simulink model "EEBL_Scenario_02_cs"  (Simulink 7.6)
settings: Solver=ode5  SolverMode=SingleTasking  StartTime=0.0  StopTime=15  FixedStep=1/100  RelTol=1e-3
model workspace (MAT data in the model file):
  mbox_table : struct (value not decoded)
  model_closed = 0
  sim_status = 0
PreLoadFcn:
  | check_NUTS_defined;
  | 
  | assignin('base',['model_closed_' bdroot],false);addpath('../includes_V2x');
InitFcn:
  | PreScanExperimentInitFcn(bdroot)
StopFcn:
  | PreScanExperimentStopFcn(bdroot)
undefined symbols (not defined in the file): acceleration, actorID, actorType, DiscIntNeverNeededParam, GPS_alt, GPS_lat, GPS_long, intmax, lightBarInUse, messageID, publicVehicleType, rotZ, sireneInUse, trafficLightPriority, turnAdvice, velocity, x_ini_VRML, y_ini_VRML, yawRate, z_ini_VRML
libraries: simulink x54, PreScanSimulinkLibrary x11, simulink_extras x8, PreScanUsefulBlocks x6, simulink_need_slupdate x1
(part 1 of 10)
CloseFcn:
  | evalin('base',['clear model_closed_' bdroot]);
  | 
  | try
  |     close (V2X_PlotSpeed)
  | end
  | 
  | try
  |     close (EEBL_PlotSpeed)
  | end
settings Model: Creator=PRESCAN  LastModifiedBy=buildbot
settings OptimizationCC: InitFltsAndDblsToZero=on
settings DebuggingCC: SaveWithParameterizedLinksMsg=none  SignalResolutionControl=TryResolveAllWithWarning  SolverPrmCheckMsg=none  MultiTaskDSMMsg=warning  MultiTaskCondExecSysMsg=none
settings SFSimCC: SimParseCustomCode=off
settings RTWCC: IncludeERTFirstTime=on
settings GRTTargetCC: TargetFcnLib=ansi_tfl_tmw.mat

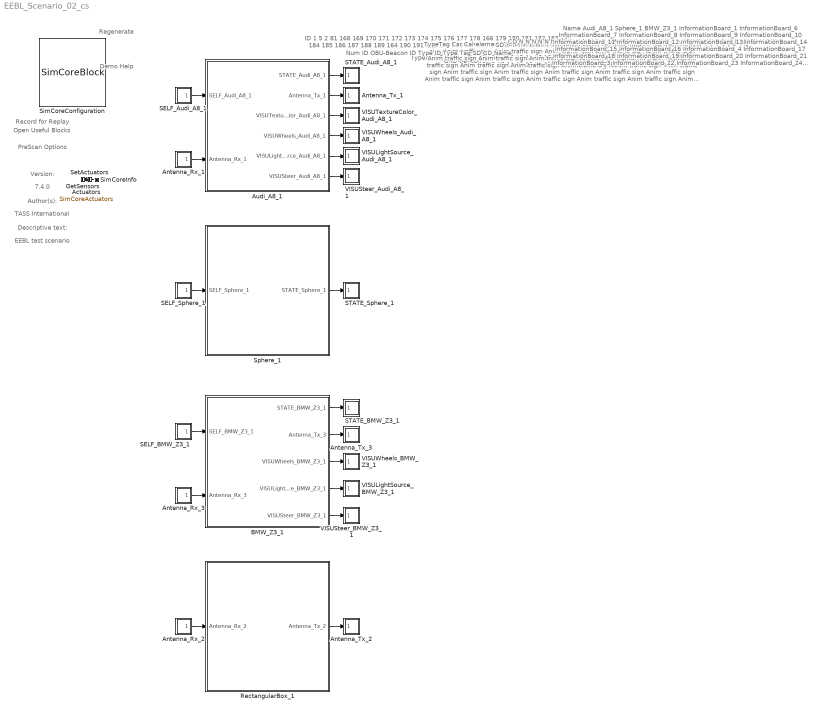
== system EEBL_Scenario_02_cs ==
  note: Demo Help
  note: Regenerate
  note: Record for Replay
  note: Open Useful Blocks
  note: PreScan Options
  note: Version:
  note: 7.4.0
  note: Author(s):
  note: TASS International
  note: Descriptive text:
  note: EEBL test scenario
  note: ID
      |
      | 1
      | 5
      | 2
      | 81
      | 168
      | 169
      | 170
      | 171
      | 172
      | 173
      | 174
      | 175
      | 176
      | 177
      | 178
      | 166
      | 179
      | 180
      | 181
      | 182
      | 183
      | 165
      | 184
      | 185
      | 186
      | 187
      | 188
      | 189
      | 164
      | 190
      | 191
      | 192
      | 193
      | 194
      | 167
      | 195
      | 196
      | 197
      | 198
      | 199
      | 200
      | 201
      | 163
  note: OBU-Beacon ID
  note: TypeID
      |
      | 1
      | 5
      | 1
      | 15
      | 15
      | 15
      | 15
      | 15
      | 15
      | 15
      | 15
      | 15
      | 15
      | 15
      | 15
      | 15
      | 15
      | 15
      | 15
      | 15
      | 15
      | 15
      | 15
      | 15
      | 15
      | 15
      | 15
      | 15
      | 15
      | 15
      | 15
      | 15
      | 15
      | 15
      | 15
      | 15
      | 15
      | 15
      | 15
      | 15
      | 15
      | 15
      | 16
  note: TypeTag
      |
      | Car
      | Cal element
      | Car
      | Anim traffic sign
      | Anim traffic sign
      | Anim traffic sign
      | Anim traffic sign
      | Anim traffic sign
      | Anim traffic sign
      | Anim traffic sign
      | Anim traffic sign
      | Anim traffic sign
      | Anim traffic sign
      | Anim traffic sign
      | Anim traffic sign
      | Anim traffic sign
      | Anim traffic sign
      | Anim traffic sign
      | Anim traffic sign
      | Anim traffic sign
      | Anim traffic sign
      | Anim traffic sign
      | Anim traffic sign
      | Anim traffic sign
      | Anim traffic sign
      | Anim traffic sign
      | Anim traffic sign
      | Anim traffic sign
      | Anim traffic sign
      | Anim traffic sign
      | Anim traffic sign
      | Anim traffic sign
      | Anim traffic sign
      | Anim traffic sign
      | Anim traffic sign
      | Anim traffic sign
      | Anim traffic sign
      | Anim traffic sign
      | Anim traffic sign
      | Anim traffic sign
      | Anim traffic sign
      | Anim traffic sign
      | Abstract object
  note: SD
      |
      | Y
      | Y
      | Y
      | Y
      | Y
      | Y
      | Y
      | Y
      | Y
      | Y
      | Y
      | Y
      | Y
      | Y
      | Y
      | Y
      | Y
      | Y
      | Y
      | Y
      | Y
      | Y
      | Y
      | Y
      | Y
      | Y
      | Y
      | Y
      | Y
      | Y
      | Y
      | Y
      | Y
      | Y
      | Y
      | Y
      | Y
      | Y
      | Y
      | Y
      | Y
      | Y
      | N
  note: CD
      |
      | N
      | N
      | N
      | N
      | N
      | N
      | N
      | N
      | N
      | N
      | N
      | N
      | N
      | N
      | N
      | N
      | N
      | N
      | N
      | N
      | N
      | N
      | N
      | N
      | N
      | N
      | N
      | N
      | N
      | N
      | N
      | N
      | N
      | N
      | N
      | N
      | N
      | N
      | N
      | N
      | N
      | N
      | N
  note: Name
      |
      | Audi_A8_1
      | Sphere_1
      | BMW_Z3_1
      | InformationBoard_1
      | InformationBoard_6
      | InformationBoard_7
      | InformationBoard_8
      | InformationBoard_9
      | InformationBoard_10
      | InformationBoard_11
      | InformationBoard_12
      | InformationBoard_13
      | InformationBoard_14
      | InformationBoard_15
      | InformationBoard_16
      | InformationBoard_4
      | InformationBoard_17
      | InformationBoard_18
      | InformationBoard_19
      | InformationBoard_20
      | InformationBoard_21
      | InformationBoard_3
      | InformationBoard_22
      | InformationBoard_23
      | InformationBoard_24
      | InformationBoard_25
      | InformationBoard_26
      | InformationBoard_27
      | InformationBoard_2
      | InformationBoard_28
      | InformationBoard_29
      | InformationBoard_30
      | InformationBoard_31
      | InformationBoard_32
      | InformationBoard_5
      | InformationBoard_33
      | InformationBoard_34
      | InformationBoard_35
      | InformationBoard_36
      | InformationBoard_37
      | InformationBoard_38
      | InformationBoard_39
      | RectangularBox_1
  note: Num ID OBU-Beacon ID Type ID Type Tag SD CD Name
  Actuators : DataStoreMemory  Tag=Actuators  DataStoreName=SimCoreActuators  InitialValue=zeros(1167,1)
      settings: DeleteFcn=PreScanBlockDeleteFcn;
  Antenna_Rx_1 : Subsystem  Tag=AntennaR  Priority=3  mask(PreScan Source Block: Antenna Receiver){Channel=1, NrEntitiesOut=2, PortName=Antenna_Rx_1, PortIndex=8, PortWidth=456, TimeStep=1/100}
      mask prompts: Channel "User Specified: Channel# [-]"; NrEntitiesOut "User Specified: # of Visible Actors"; PortName "Auto Assigned: Port Name [-]"; PortIndex "Auto Assigned: Index [-]"; PortWidth "Auto Assigned: Port Dimensions [-]"; TimeStep "Auto Assigned: Upload Period [s]"
      mask help:
      | Using the Antenna Receiver (RX) and Transmitter (TX) information between actors can be exchanged. This is done over a channel number to be specified by the user.
      |
      | The Antenna Reciever receives actor information and user-definable signals.
      |
      | For more information, please click Help.
      settings: DeleteFcn=PreScanBlockDeleteFcn;
      mask Help: eval('openHelp(424)')
      mask Display: image(imread('Rx.png'))
  Antenna_Rx_2 : Subsystem  Tag=AntennaR  Priority=3  mask(PreScan Source Block: Antenna Receiver){Channel=1, NrEntitiesOut=2, PortName=Antenna_Rx_2, PortIndex=936, PortWidth=456, TimeStep=1/100}
      mask prompts: Channel "User Specified: Channel# [-]"; NrEntitiesOut "User Specified: # of Visible Actors"; PortName "Auto Assigned: Port Name [-]"; PortIndex "Auto Assigned: Index [-]"; PortWidth "Auto Assigned: Port Dimensions [-]"; TimeStep "Auto Assigned: Upload Period [s]"
      mask help:
      | Using the Antenna Receiver (RX) and Transmitter (TX) information between actors can be exchanged. This is done over a channel number to be specified by the user.
      |
      | The Antenna Reciever receives actor information and user-definable signals.
      |
      | For more information, please click Help.
      settings: DeleteFcn=PreScanBlockDeleteFcn;
      mask Help: eval('openHelp(424)')
      mask Display: image(imread('Rx.png'))
  Antenna_Rx_3 : Subsystem  Tag=AntennaR  Priority=3  mask(PreScan Source Block: Antenna Receiver){Channel=1, NrEntitiesOut=2, PortName=Antenna_Rx_3, PortIndex=480, PortWidth=456, TimeStep=1/100}
      mask prompts: Channel "User Specified: Channel# [-]"; NrEntitiesOut "User Specified: # of Visible Actors"; PortName "Auto Assigned: Port Name [-]"; PortIndex "Auto Assigned: Index [-]"; PortWidth "Auto Assigned: Port Dimensions [-]"; TimeStep "Auto Assigned: Upload Period [s]"
      mask help:
      | Using the Antenna Receiver (RX) and Transmitter (TX) information between actors can be exchanged. This is done over a channel number to be specified by the user.
      |
      | The Antenna Reciever receives actor information and user-definable signals.
      |
      | For more information, please click Help.
      settings: DeleteFcn=PreScanBlockDeleteFcn;
      mask Help: eval('openHelp(424)')
      mask Display: image(imread('Rx.png'))
  Antenna_Tx_1 : Subsystem  Tag=AntennaT  Priority=0  mask(PreScan Sink Block: AntennaT){Channel=1, PortName=Antenna_Tx_1, PortIndex=15, PortWidth=205, TimeStep=1/100}
      mask prompts: Channel "User Specified: Channel# [-]"; PortName "Auto Assigned: Port Name [-]"; PortIndex "Auto Assigned: Index [-]"; PortWidth "Auto Assigned: Port Dimensions [-]"; TimeStep "Auto Assigned: Upload Period [s]"
      mask help:
      | Using the Antenna Receiver (RX) and Transmitter (TX) information between actors can be exchanged. This is done over a channel number to be specified by the user.
      |
      | The Antenna Transmitter contains the following, user-definable signals:
      |
      | - Warning Signal ID	[-]
      | - Maneuvre ID		[-]
      | - Vehicle Type 		[-]
      | - Braking Capacity	[-]
      | - Vehicle Size		[-]
      | - Spares (1:10)		[-]
      |
      | For more information, please click Help.
      settings: DeleteFcn=PreScanBlockDeleteFcn;
      mask Help: eval('openHelp(424)')
      mask Display: image(imread('Tx.png'))
  Antenna_Tx_2 : Subsystem  Tag=AntennaT  Priority=0  mask(PreScan Sink Block: AntennaT){Channel=1, PortName=Antenna_Tx_2, PortIndex=962, PortWidth=205, TimeStep=1/100}
      mask prompts: Channel "User Specified: Channel# [-]"; PortName "Auto Assigned: Port Name [-]"; PortIndex "Auto Assigned: Index [-]"; PortWidth "Auto Assigned: Port Dimensions [-]"; TimeStep "Auto Assigned: Upload Period [s]"
      mask help:
      | Using the Antenna Receiver (RX) and Transmitter (TX) information between actors can be exchanged. This is done over a channel number to be specified by the user.
      |
      | The Antenna Transmitter contains the following, user-definable signals:
      |
      | - Warning Signal ID	[-]
      | - Maneuvre ID		[-]
      | - Vehicle Type 		[-]
      | - Braking Capacity	[-]
      | - Vehicle Size		[-]
      | - Spares (1:10)		[-]
      |
      | For more information, please click Help.
      settings: DeleteFcn=PreScanBlockDeleteFcn;
      mask Help: eval('openHelp(424)')
      mask Display: image(imread('Tx.png'))
  Antenna_Tx_3 : Subsystem  Tag=AntennaT  Priority=0  mask(PreScan Sink Block: AntennaT){Channel=1, PortName=Antenna_Tx_3, PortIndex=481, PortWidth=205, TimeStep=1/100}
      mask prompts: Channel "User Specified: Channel# [-]"; PortName "Auto Assigned: Port Name [-]"; PortIndex "Auto Assigned: Index [-]"; PortWidth "Auto Assigned: Port Dimensions [-]"; TimeStep "Auto Assigned: Upload Period [s]"
      mask help:
      | Using the Antenna Receiver (RX) and Transmitter (TX) information between actors can be exchanged. This is done over a channel number to be specified by the user.
      |
      | The Antenna Transmitter contains the following, user-definable signals:
      |
      | - Warning Signal ID	[-]
      | - Maneuvre ID		[-]
      | - Vehicle Type 		[-]
      | - Braking Capacity	[-]
      | - Vehicle Size		[-]
      | - Spares (1:10)		[-]
      |
      | For more information, please click Help.
      settings: DeleteFcn=PreScanBlockDeleteFcn;
      mask Help: eval('openHelp(424)')
      mask Display: image(imread('Tx.png'))
  Audi_A8_1 : Subsystem  Tag=WorldObjectSubSystem  InitFcn=UniqueId = '13';
      mask Display: image(imread('Audi_A8.jpg'));color('white');text(0,0,' ID=1\n')
  BMW_Z3_1 : Subsystem  Tag=WorldObjectSubSystem  InitFcn=UniqueId = '205';
      mask Display: image(imread('BMW_Z3.jpg'));color('white');text(0,0,' ID=2\n')
  GetSensors : Subsystem  Tag=GetSensors  Priority=2  mask(PreScan Simulation Core Block){NrOfSensors=1392, TimeStep=1/100}
      mask prompts: NrOfSensors "Number of sensor values"; TimeStep "Timestep [s]"
      mask help:
      | Please do not remove this block from the PreScan compilation sheet,
      | as it contains essential configuration parameters for a PreScan simulation.
      settings: DeleteFcn=PreScanBlockDeleteFcn;
  RectangularBox_1 : Subsystem  Tag=WorldObjectSubSystem  InitFcn=UniqueId = '557';
      mask Display: image(imread('RectangularBox.jpg'));color('white');text(0,0,' ID=163\n')
  SELF_Audi_A8_1 : Subsystem  Tag=SELF  Priority=3  mask(PreScan Source Block: SELF){PortName=SELF_Audi_A8_1, PortIndex=0, PortWidth=8, TimeStep=1/100}
      mask prompts: PortName "Auto-Assigned: Port Name [-]"; PortIndex "Auto-Assigned: Port Index [-]"; PortWidth "Auto-Assigned: Port Dimensions"; TimeStep "Auto-Assigned: Upload Period [s]"
      mask help:
      | The SELF port shows (state) information of the actor itself. The outputs are position in the experiment's axis system and the GPS coordinates, and the object's absolute velocity and compass heading.
      |
      | For more information, please click Help.
      settings: DeleteFcn=PreScanBlockDeleteFcn;
      mask Help: eval('openHelp(462)')
      mask Display: image(imread('GPS.png'))
  SELF_BMW_Z3_1 : Subsystem  Tag=SELF  Priority=3  mask(PreScan Source Block: SELF){PortName=SELF_BMW_Z3_1, PortIndex=472, PortWidth=8, TimeStep=1/100}
      mask prompts: PortName "Auto-Assigned: Port Name [-]"; PortIndex "Auto-Assigned: Port Index [-]"; PortWidth "Auto-Assigned: Port Dimensions"; TimeStep "Auto-Assigned: Upload Period [s]"
      mask help:
      | The SELF port shows (state) information of the actor itself. The outputs are position in the experiment's axis system and the GPS coordinates, and the object's absolute velocity and compass heading.
      |
      | For more information, please click Help.
      settings: DeleteFcn=PreScanBlockDeleteFcn;
      mask Help: eval('openHelp(462)')
      mask Display: image(imread('GPS.png'))
  SELF_Sphere_1 : Subsystem  Tag=SELF  Priority=3  mask(PreScan Source Block: SELF){PortName=SELF_Sphere_1, PortIndex=464, PortWidth=8, TimeStep=1/100}
      mask prompts: PortName "Auto-Assigned: Port Name [-]"; PortIndex "Auto-Assigned: Port Index [-]"; PortWidth "Auto-Assigned: Port Dimensions"; TimeStep "Auto-Assigned: Upload Period [s]"
      mask help:
      | The SELF port shows (state) information of the actor itself. The outputs are position in the experiment's axis system and the GPS coordinates, and the object's absolute velocity and compass heading.
      |
      | For more information, please click Help.
      settings: DeleteFcn=PreScanBlockDeleteFcn;
      mask Help: eval('openHelp(462)')
      mask Display: image(imread('GPS.png'))
  STATE_Audi_A8_1 : Subsystem  Tag=State  Priority=0  mask(PreScan Sink Block: State){x0=-2.0003382369952085, y0=3.5736286855864789, z0=0.55, Roll0=0, Pitch0=0, Yaw0=0.92319780373458116, TimeStep=1/100}
      mask prompts: x0 "Ini x-position VEHICLE wrt GLOBAL axis system [m]"; y0 "Ini y-position VEHICLE wrt GLOBAL axis system [m]"; z0 "Ini z-position VEHICLE wrt GLOBAL axis system [m]"; Roll0 "Ini roll-angle BODY wrt VEHICLE axis system [deg]"; Pitch0 "Ini pitch-angle BODY wrt VEHICLE axis system [deg]"; Yaw0 "Ini yaw-angle VEHICLE wrt GLOBAL axis system [deg]"; TimeStep "Time Step [s]"
      mask help:
      | The Actor State contains a vector signal of size (9x1), containing the following signals:
      |
      | -  Position                  (x,y,z)                                     [m]
      | -  Velocity                  (vx,vy,vz)                               [m/s]
      | -  Angles                    (Roll, Pitch, Yaw)                   [rad]
      |
      | The Actor state is defined in the global axis system.
      | The state is superponed on the Initial position defined in the GUI.
      |
      | For more information, please click Help.
      settings: DeleteFcn=PreScanBlockDeleteFcn;
      mask Help: eval('openHelp(222)')
      mask Display: image(imread('State.png'))
  STATE_BMW_Z3_1 : Subsystem  Tag=State  Priority=0  mask(PreScan Sink Block: State){x0=59.766689592078251, y0=8.4452137651818937, z0=0.69, Roll0=0, Pitch0=0, Yaw0=8.0780561606359811, TimeStep=1/100}
      mask prompts: x0 "Ini x-position VEHICLE wrt GLOBAL axis system [m]"; y0 "Ini y-position VEHICLE wrt GLOBAL axis system [m]"; z0 "Ini z-position VEHICLE wrt GLOBAL axis system [m]"; Roll0 "Ini roll-angle BODY wrt VEHICLE axis system [deg]"; Pitch0 "Ini pitch-angle BODY wrt VEHICLE axis system [deg]"; Yaw0 "Ini yaw-angle VEHICLE wrt GLOBAL axis system [deg]"; TimeStep "Time Step [s]"
      mask help:
      | The Actor State contains a vector signal of size (9x1), containing the following signals:
      |
      | -  Position                  (x,y,z)                                     [m]
      | -  Velocity                  (vx,vy,vz)                               [m/s]
      | -  Angles                    (Roll, Pitch, Yaw)                   [rad]
      |
      | The Actor state is defined in the global axis system.
      | The state is superponed on the Initial position defined in the GUI.
      |
      | For more information, please click Help.
      settings: DeleteFcn=PreScanBlockDeleteFcn;
      mask Help: eval('openHelp(222)')
      mask Display: image(imread('State.png'))
  STATE_Sphere_1 : Subsystem  Tag=State  Priority=0  mask(PreScan Sink Block: State){x0=-2.0003746851196036, y0=3.5683845581685842, z0=0, Roll0=0, Pitch0=0, Yaw0=0.65951613396799758, TimeStep=1/100}
      mask prompts: x0 "Ini x-position VEHICLE wrt GLOBAL axis system [m]"; y0 "Ini y-position VEHICLE wrt GLOBAL axis system [m]"; z0 "Ini z-position VEHICLE wrt GLOBAL axis system [m]"; Roll0 "Ini roll-angle BODY wrt VEHICLE axis system [deg]"; Pitch0 "Ini pitch-angle BODY wrt VEHICLE axis system [deg]"; Yaw0 "Ini yaw-angle VEHICLE wrt GLOBAL axis system [deg]"; TimeStep "Time Step [s]"
      mask help:
      | The Actor State contains a vector signal of size (9x1), containing the following signals:
      |
      | -  Position                  (x,y,z)                                     [m]
      | -  Velocity                  (vx,vy,vz)                               [m/s]
      | -  Angles                    (Roll, Pitch, Yaw)                   [rad]
      |
      | The Actor state is defined in the global axis system.
      | The state is superponed on the Initial position defined in the GUI.
      |
      | For more information, please click Help.
      settings: DeleteFcn=PreScanBlockDeleteFcn;
      mask Help: eval('openHelp(222)')
      mask Display: image(imread('State.png'))
  SetActuators : Subsystem  Tag=SetActuators  Priority=1  mask(PreScan Simulation Core Block){TimeStep=1/100, NrOfActuators=1167}
      mask prompts: TimeStep "Timestep [s]"; NrOfActuators "Number of actuator values"
      mask help:
      | Please do not remove this block from the PreScan compilation sheet,
      | as it contains essential configuration parameters for a PreScan simulation.
      settings: DeleteFcn=PreScanBlockDeleteFcn;
  SimCoreConfiguration : M-S-Function  Tag=SimCoreConfiguration  Description=7554E7A75508BA4AB74C9CE496844D0A64444FB1F4C419A76FFCA00764D87D8D  FunctionName=SimCoreBlock  Parameters=ExperimentXML PortsXML SimulationCore HostName CheckStart EnableLog RfR EnableGPUAccel ShowComputationTime  mask(PreScan Simulation Core Configurator){SimulationCore=NUTS, HostName=0, CheckStart=0, prescanversion='7.4.0', EnableLog=off, RfR=0, EnableGPUAccel=off, ShowComputationTime=off}
      mask prompts: SimulationCore "Simulation Core"; HostName "Simulation Host"; CheckStart "Show START Dialog"; prescanversion "PreScan Version"; EnableLog "Create TA Log"; RfR "Record for Replay"; EnableGPUAccel "Enable GPU Acceleration"; ShowComputationTime "Show ComputationTime Scope"
      mask help:
      | Please do not remove this block from the PreScan compilation sheet,
      | as it contains essential configuration parameter for a PreScan simulation.
      mask init:
      | model = bdroot;
      | ExperimentXML = [model(1:end-3) '.pex'];
      | PortsXML = [model '_ports.pcd'];
      settings: DeleteFcn=PreScanBlockDeleteFcn;  ModelCloseFcn=assignin('base',['model_closed_' bdroot],true);
      mask Help: eval('openHelp(812)')
      mask Display: image(imread('prescanlogo.ico'))
  SimCoreInfo : Subsystem  Tag=SimCoreInfo
  Sphere_1 : Subsystem  Tag=WorldObjectSubSystem  InitFcn=UniqueId = '36';
      mask Display: image(imread('Sphere.jpg'));color('white');text(0,0,' ID=5\n')
  VISULightSource_Audi_A8_1 : Subsystem  Tag=VisuLightSource  Priority=0
      settings: DeleteFcn=PreScanBlockDeleteFcn;
      mask Type: PreScan Sink Block: VisuLightSource
      mask Description:
      | The VisuLightSource block provides a way to animate Light Sources of the indicator, braking, fog and main lights of a vehicle.
      | 
      | For more information, please click Help.
      mask Help: eval('openHelp(223)')
      mask Display: image(imread('RearLight.png'))
  VISULightSource_BMW_Z3_1 : Subsystem  Tag=VisuLightSource  Priority=0
      settings: DeleteFcn=PreScanBlockDeleteFcn;
      mask Type: PreScan Sink Block: VisuLightSource
      mask Description:
      | The VisuLightSource block provides a way to animate Light Sources of the indicator, braking, fog and main lights of a vehicle.
      | 
      | For more information, please click Help.
      mask Help: eval('openHelp(223)')
      mask Display: image(imread('RearLight.png'))
  VISUSteer_Audi_A8_1 : Subsystem  Tag=VisuSteer  Priority=0
      settings: DeleteFcn=PreScanBlockDeleteFcn;
      mask Type: PreScan Sink Block: VisuSteer
      mask Description:
      | The VisuSteer block provides a way to adapt the orientation of the steering column and steering wheel of a vehicle.
      | 
      | For more information, please click Help.
      mask Help: eval('openHelp(223)')
      mask Display: image(imread('steeringwheel.png'))
  VISUSteer_BMW_Z3_1 : Subsystem  Tag=VisuSteer  Priority=0
      settings: DeleteFcn=PreScanBlockDeleteFcn;
      mask Type: PreScan Sink Block: VisuSteer
      mask Description:
      | The VisuSteer block provides a way to adapt the orientation of the steering column and steering wheel of a vehicle.
      | 
      | For more information, please click Help.
      mask Help: eval('openHelp(223)')
      mask Display: image(imread('steeringwheel.png'))
  VISUTextureColor_Audi_A8_1 : Subsystem  Tag=VisuTextureColor  Priority=0
      settings: DeleteFcn=PreScanBlockDeleteFcn;
      mask Type: PreScan Sink Block: VisuTextureColor
      mask Description:
      | The Texture Color block provides a way to adapt the color of a vehicle.
      | 
      | For more information, please click Help.
      mask Help: eval('openHelp(230)')
      mask Display: image(imread('TextureColor.png'))
  VISUWheels_Audi_A8_1 : Subsystem  Tag=VisuWheels  Priority=0
      settings: DeleteFcn=PreScanBlockDeleteFcn;
      mask Type: PreScan Sink Block: VisuWheels
      mask Description:
      | The VisuWheels block provides a way to animate the wheels of a vehicle, with steering, rotation (because of velocity) and z-displacement.
      | 
      | For more information, please click Help.
      mask Help: eval('openHelp(223)')
      mask Display: image(imread('wheel.png'))
  VISUWheels_BMW_Z3_1 : Subsystem  Tag=VisuWheels  Priority=0
      settings: DeleteFcn=PreScanBlockDeleteFcn;
      mask Type: PreScan Sink Block: VisuWheels
      mask Description:
      | The VisuWheels block provides a way to animate the wheels of a vehicle, with steering, rotation (because of velocity) and z-displacement.
      | 
      | For more information, please click Help.
      mask Help: eval('openHelp(223)')
      mask Display: image(imread('wheel.png'))
  wires:
  Audi_A8_1/1(STATE_Audi_A8_1) -> STATE_Audi_A8_1/1(State)
  SELF_Audi_A8_1/1(U) -> Audi_A8_1/1(SELF_Audi_A8_1)
  Antenna_Rx_1/1(U) -> Audi_A8_1/2(Antenna_Rx_1)
  Audi_A8_1/2(Antenna_Tx_1) -> Antenna_Tx_1/1(Y)
  Audi_A8_1/3(VISUTextureColor_Audi_A8_1) -> VISUTextureColor_Audi_A8_1/1(TextureColor)
  Audi_A8_1/4(VISUWheels_Audi_A8_1) -> VISUWheels_Audi_A8_1/1(Wheels)
  Audi_A8_1/5(VISULightSource_Audi_A8_1) -> VISULightSource_Audi_A8_1/1(Lights)
  Audi_A8_1/6(VISUSteer_Audi_A8_1) -> VISUSteer_Audi_A8_1/1(Steer)
  Sphere_1/1(STATE_Sphere_1) -> STATE_Sphere_1/1(State)
  SELF_Sphere_1/1(U) -> Sphere_1/1(SELF_Sphere_1)
  BMW_Z3_1/1(STATE_BMW_Z3_1) -> STATE_BMW_Z3_1/1(State)
  SELF_BMW_Z3_1/1(U) -> BMW_Z3_1/1(SELF_BMW_Z3_1)
  Antenna_Rx_3/1(U) -> BMW_Z3_1/2(Antenna_Rx_3)
  BMW_Z3_1/2(Antenna_Tx_3) -> Antenna_Tx_3/1(Y)
  BMW_Z3_1/3(VISUWheels_BMW_Z3_1) -> VISUWheels_BMW_Z3_1/1(Wheels)
  BMW_Z3_1/4(VISULightSource_BMW_Z3_1) -> VISULightSource_BMW_Z3_1/1(Lights)
  BMW_Z3_1/5(VISUSteer_BMW_Z3_1) -> VISUSteer_BMW_Z3_1/1(Steer)
  Antenna_Rx_2/1(U) -> RectangularBox_1/1(Antenna_Rx_2)
  RectangularBox_1/1(Antenna_Tx_2) -> Antenna_Tx_2/1(Y)
  SetActuators/1(dummy) -> GetSensors/1(dummy)

== system EEBL_Scenario_02_cs/Antenna_Rx_1 ==
  Selector : Selector  IndexMode=Zero-based  IndexOptions=Starting index (dialog)  Indices=PortIndex  OutputSizes=PortWidth(1)
  U : Outport
  wires:
  Selector/1 -> U/1
  [SimCoreSensors] -> Selector/1

== system EEBL_Scenario_02_cs/Antenna_Rx_2 ==
  Selector : Selector  IndexMode=Zero-based  IndexOptions=Starting index (dialog)  Indices=PortIndex  OutputSizes=PortWidth(1)
  U : Outport
  wires:
  Selector/1 -> U/1
  [SimCoreSensors] -> Selector/1

== system EEBL_Scenario_02_cs/Antenna_Rx_3 ==
  Selector : Selector  IndexMode=Zero-based  IndexOptions=Starting index (dialog)  Indices=PortIndex  OutputSizes=PortWidth(1)
  U : Outport
  wires:
  Selector/1 -> U/1
  [SimCoreSensors] -> Selector/1

== system EEBL_Scenario_02_cs/Antenna_Tx_1 ==
  Y : Inport
  Assignment : Assignment  IndexMode=Zero-based  SampleTime=TimeStep  IndexOptions=Starting index (dialog)  Indices=PortIndex  OutputSizes=[1 1]
  Data Store Read : DataStoreRead  DataStoreName=SimCoreActuators  SampleTime=TimeStep
  Data Store Write : DataStoreWrite  DataStoreName=SimCoreActuators
  wires:
  Assignment/1 -> Data Store Write/1
  Data Store Read/1 -> Assignment/1
  Y/1 -> Assignment/2

== system EEBL_Scenario_02_cs/Antenna_Tx_2 ==
  Y : Inport
  Assignment : Assignment  IndexMode=Zero-based  SampleTime=TimeStep  IndexOptions=Starting index (dialog)  Indices=PortIndex  OutputSizes=[1 1]
  Data Store Read : DataStoreRead  DataStoreName=SimCoreActuators  SampleTime=TimeStep
  Data Store Write : DataStoreWrite  DataStoreName=SimCoreActuators
  wires:
  Assignment/1 -> Data Store Write/1
  Data Store Read/1 -> Assignment/1
  Y/1 -> Assignment/2

== system EEBL_Scenario_02_cs/Antenna_Tx_3 ==
  Y : Inport
  Assignment : Assignment  IndexMode=Zero-based  SampleTime=TimeStep  IndexOptions=Starting index (dialog)  Indices=PortIndex  OutputSizes=[1 1]
  Data Store Read : DataStoreRead  DataStoreName=SimCoreActuators  SampleTime=TimeStep
  Data Store Write : DataStoreWrite  DataStoreName=SimCoreActuators
  wires:
  Assignment/1 -> Data Store Write/1
  Data Store Read/1 -> Assignment/1
  Y/1 -> Assignment/2

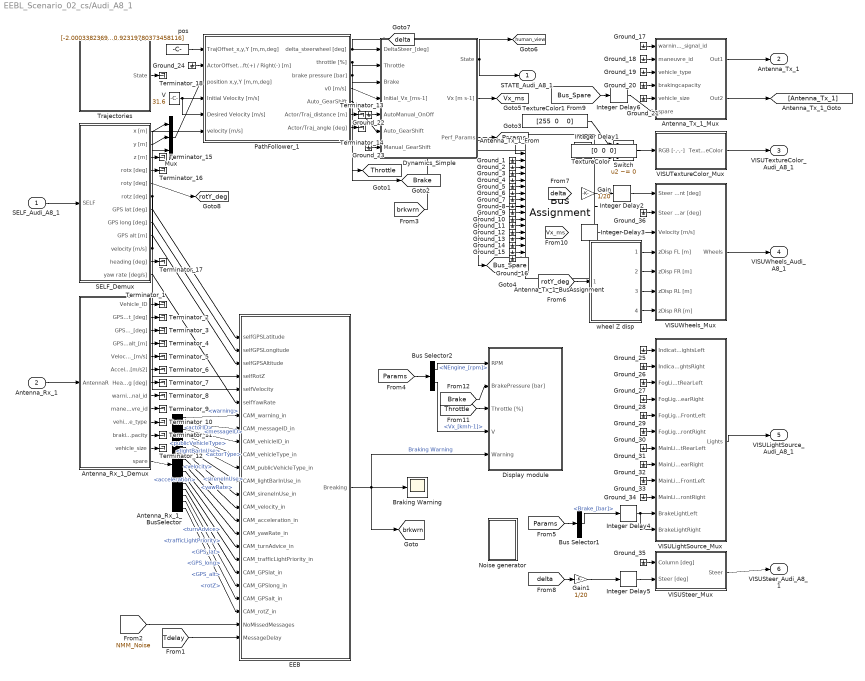
== system EEBL_Scenario_02_cs/Audi_A8_1 ==
  SELF_Audi_A8_1 : Inport  Tag=SELFInport
  Antenna_Rx_1 : Inport  Tag=AntennaRInport  Port=2
  Antenna_Rx_1_BusSelector : BusSelector  Tag=BusAntennaR  OutputSignals=warning,messageID,actorID,actorType,publicVehicleType,lightBarInUse,sireneInUse,velocity,acceleration,yawRate,turnAdvice,trafficLightPriority,GPS_lat,GPS_long,GPS_alt,rotZ
  Antenna_Rx_1_Demux : Subsystem  Tag=DemuxAntennaR  mask(PreScan Demux Block:){Channel=1}
      settings: DeleteFcn=PreScanBlockDeleteFcn;
      mask Display:
      | fprintf('Channel: %d',Channel)
      | port_label('output', 1, 'Vehicle_ID')
      | port_label('output', 2, 'GPS Pos Lat [deg]')
      | port_label('output', 3, 'GPS Pos Long [deg]')
      | port_label('output', 4, 'GPS Pos Alt [m]')
      | port_label('output', 5, 'Velocity [m/s]')
      | port_label('output', 6, 'Acceleration [m/s2]')
      | port_label('output', 7, 'Heading [deg]')
      | port_label('output', 8, 'Warning signal ID')
      | port_label('output', 9, 'Maneuvre ID')
      | port_label('output', 10, 'Vehicle Type')
      | port_label('output', 11, 'Braking Capacity')
      | port_label('output', 12, 'Vehicle Size')
      | port_label('output', 13, 'Spare')
  Antenna_Tx_1_BusAssignment : BusAssignment  Tag=BusAntennaT  AssignedSignals=warning,messageID,actorID,actorType,publicVehicleType,lightBarInUse,sireneInUse,velocity,acceleration,yawRate,turnAdvice,trafficLightPriority,GPS_lat,GPS_long,GPS_alt,rotZ
  Antenna_Tx_1_Mux : Subsystem  Tag=MuxAntennaT  mask(PreScan Mux Block:){Channel=1, TimeStep=1/100}
      mask prompts: TimeStep "Time Step [s]"
      settings: DeleteFcn=PreScanBlockDeleteFcn;
      mask Display:
      | fprintf('Channel: %d',Channel)
      | port_label('input', 1, 'Warning signal ID')
      | port_label('input', 2, 'Maneuvre ID')
      | port_label('input', 3, 'Vehicle Type')
      | port_label('input', 4, 'Braking Capacity')
      | port_label('input', 5, 'Vehicle Size')
      | port_label('input', 6, 'spare')
  Braking Warning : Scope
      settings: SaveName=ScopeData2
  Bus Selector1 : BusSelector  OutputSignals=Brake_[bar]
  Bus Selector2 : BusSelector  OutputSignals=NEngine_[rpm],Vx_[kmh-1]
  Display module : Subsystem  mask{DisplaySwitch=on, DisplayFreq=25}
      mask prompts: DisplaySwitch "Dispaly"; DisplayFreq "Display Frequency"
  Dynamics_Simple : Subsystem  Tag=Simple_Vehicle_Dynamics  mask(PreScan Block: Simple Dynamics){Migrate=off, TimeStep=1/100, ComputationMode=Continuous_Time}
      mask prompts: Migrate "Migrate. During migration this block will be replaced by a newer one."; TimeStep "Auto assigned: Time Step [s]"; ComputationMode "Computation mode:"
      mask help:
      | The Simple Dynamics Model is selected in the GUI to simulate vehicle dynamics behavior.
      |
      | The Simple Dynamics Model is completely open to the user. The parameters of this model can be set in the Simple Dynamics dialog in the GUI.
      |
      | For more information, please click Help.
      mask init:
      | p = SimpleDyn_pars;
      settings: DeleteFcn=PreScanBlockDeleteFcn;
      mask Help: eval('openHelp(220)')
      mask Display:
      | image(imread('SimpleDyn.png'))
      | port_label('input', 1, '{\delta}_S_t_ _e_e_r [deg]','texmode','on')
      | port_label('input', 2, 'Throttle [%]')
      | port_label('input', 3, 'Brake Pres [bar]')
      | port_label('input', 4, 'V_0 [ms-1]','texmode','on')
      | port_label('input', 5, 'Auto=[0]/Manual=[1]')
      | port_label('input', 6, 'Auto_GearShift')
      | port_label('input', 7, 'Manual_GearShift')
      | port_label('output', 1, 'State')
      | port_label('output', 2, 'Vx [ms-1]')
      | port_label('output', 3, 'Perf Params')
  EEB : Subsystem
  Gain : Gain  Gain=1/20
  Gain1 : Gain  Gain=1/20
  Ground_{1..36} (36 alike) : Ground
  Integer Delay{1..6} (6 alike) : simulink/Discrete/Integer Delay  NumDelays=1  InputProcessing=Inherited  vinit=0.0  samptime=-1
  Mux : Mux  Inputs=3
  Noise generator : Subsystem
  PathFollower_1 : Subsystem  Tag=pathFollower  mask(PreScan Block: Path Follower){Migrate=on, FileName='Trajectory_1.mat', TunableSteeringGain=1, XShifting_wrt_COG=0}
      mask prompts: Migrate "Migrate. During migration this block will be replaced by a newer one."; FileName "Trajectory Name"; TunableSteeringGain "TunableSteeringGain [-]"; XShifting_wrt_COG "XShifting_wrt_COG [m]"
      mask help:
      | The Path Follower Model is selected in the GUI to simulate driver behavior.
      |
      | For more information, please click Help.
      mask init:
      | load(['trajectories/',eval(FileName)])
      | traject=trajectory';
      | 
      | Traj_x=traject(:,2);
      | Traj_y=traject(:,3);
      | Traj_z=traject(:,4);
      | Traj_vx=traject(:,8);
      | Traj_vy=traject(:,9);
      | Traj_vz=traject(:,10);
      mask Help: eval('openHelp(232)')
  SELF_Demux : Subsystem  Tag=DemuxSELF
      settings: DeleteFcn=PreScanBlockDeleteFcn;
      mask Type: PreScan Demux Block:
      mask Display:
      | port_label('output',1,'x [m]')
      | port_label('output',2,'y [m]')
      | port_label('output',3,'z [m]','texmode','on')
      | port_label('output',4,'Rotx [deg]','texmode','on')
      | port_label('output',5,'Roty [deg]','texmode','on')
      | port_label('output',6,'Rotz [deg]','texmode','on')
      | port_label('output',7,'GPS lat [deg]','texmode','on')
      | port_label('output',8,'GPS long [deg]','texmode','on')
      | port_label('output',9,'GPS alt [m]','texmode','on')
      | port_label('output',10,'Velocity [m/s]')
      | port_label('output',11,'Heading [deg]')
      | port_label('output',12,'Yaw rate [deg/s]')
  Switch : Switch  Criteria=u2 ~= 0
  Terminator_{1..18} (18 alike) : Terminator
  TextureColor : Constant  Tag=TextureColor  Value="[0  0  0]"
  TextureColor1 : Constant  Tag=TextureColor  Value="[255  0    0]"
  Trajectories : Subsystem  Tag=Trajectories
      settings: DeleteFcn=PreScanBlockDeleteFcn;
      mask Type: PreScan Source Block: Trajectories
      mask Description:
      | The Trajectory block contains the trajectories defined in the PreScan Experiment Editor. The output of the trajectory block is the (vehicle) State.
      | 
      | For more information, please click Help.
      mask Help: eval('openHelp(312)')
      mask Display: image(imread('Trajectory.png'));
  V : Constant  Value=31.6
  VISULightSource_Mux : Subsystem  Tag=MuxLightSource
      settings: DeleteFcn=PreScanBlockDeleteFcn;
      mask Type: PreScan Mux Block:
  VISUSteer_Mux : Subsystem  Tag=MuxSteer
      settings: DeleteFcn=PreScanBlockDeleteFcn;
      mask Type: PreScan Mux Block:
  VISUTextureColor_Mux : Subsystem  Tag=MuxSteer
      settings: DeleteFcn=PreScanBlockDeleteFcn;
      mask Type: PreScan Mux Block:
  VISUWheels_Mux : Subsystem  Tag=MuxWheels  mask(PreScan Mux Block:){TimeStep=1/100}
      mask prompts: TimeStep "Auto Assigned: Time Step [s]"
      settings: DeleteFcn=PreScanBlockDeleteFcn;
  pos : Constant  Tag=pos  Value=[-2.0003382369952085 3.5736286855864789 0.92319780373458116]
  wheel Z disp : Subsystem  mask(Simple Dynamics parameters){a=1.17, b=1.77}
      mask prompts: a "Distance to the front wheel from cars center of gravity a [m]"; b "Distance to the back wheel from cars center of gravity b [m]"
  STATE_Audi_A8_1 : Outport  Tag=StateOutport
  Antenna_Tx_1 : Outport  Tag=AntennaTOutport  Port=2
  VISUTextureColor_Audi_A8_1 : Outport  Tag=VisuTextureColorOutport  Port=3  SampleTime=1/100
  VISUWheels_Audi_A8_1 : Outport  Tag=VisuWheelsOutport  Port=4  SampleTime=1/100
  VISULightSource_Audi_A8_1 : Outport  Tag=VisuLightsOutport  Port=5  SampleTime=1/100
  VISUSteer_Audi_A8_1 : Outport  Tag=VisuSteerOutport  Port=6  SampleTime=1/100
  tag scope: Brake=global, Bus_Spare=global, Params=global, Throttle=global, Vx_ms=global, brkwrn=global, delta=global, human_view=global, rotY_deg=global
  wires:
  [delta] -> Gain/1
  [rotY_deg] -> wheel Z disp/1(rotY [deg])
  [NMM_Noise] -> EEB/23(NoMissedMessages)
  [Tdelay] -> EEB/24(MessageDelay)
  EEB/1(Breaking) -> Braking Warning/1, [brkwrn], Display module/5(Warning)  "Braking Warning"
  [brkwrn] -> Integer Delay1/1
  Gain/1 -> Integer Delay2/1
  [Bus_Spare] -> Integer Delay6/1
  Integer Delay1/1 -> Switch/2
  [Vx_ms] -> Integer Delay3/1
  [delta] -> Gain1/1
  Bus Selector1/1 -> Integer Delay4/1  "<Brake_[bar]>"
  Gain1/1 -> Integer Delay5/1
  [Params] -> Bus Selector1/1
  Bus Selector2/1 -> Display module/1(RPM)  "<NEngine_[rpm]>"
  Bus Selector2/2 -> Display module/4(V)  "<Vx_[kmh-1]>"
  [Params] -> Bus Selector2/1
  [Throttle] -> Display module/3(Throttle [%])
  [Brake] -> Display module/2(BrakePressure [bar])
  pos/1 -> PathFollower_1/1(TrajOffset_x,y,Y [m,m,deg])
  SELF_Audi_A8_1/1 -> SELF_Demux/1(SELF)
  Antenna_Rx_1_Demux/13(spare) -> Antenna_Rx_1_BusSelector/1
  Antenna_Rx_1/1 -> Antenna_Rx_1_Demux/1(AntennaR)
  Antenna_Tx_1_Mux/2(Out2) -> [Antenna_Tx_1]
  [Antenna_Tx_1] -> Antenna_Tx_1_BusAssignment/1
  Antenna_Tx_1_Mux/1(Out1) -> Antenna_Tx_1/1
  VISUTextureColor_Mux/1(TextureColor) -> VISUTextureColor_Audi_A8_1/1
  TextureColor/1 -> Switch/3
  VISUWheels_Mux/1(Wheels) -> VISUWheels_Audi_A8_1/1
  VISULightSource_Mux/1(Lights) -> VISULightSource_Audi_A8_1/1
  VISUSteer_Mux/1(Steer) -> VISUSteer_Audi_A8_1/1
  Dynamics_Simple/2(Vx [m s-1]) -> [Vx_ms]
  PathFollower_1/4(v0 [m/s]) -> Dynamics_Simple/4(Initial_Vx_[ms-1])
  PathFollower_1/5(Auto_GearShift) -> Dynamics_Simple/6(Auto_GearShift)
  PathFollower_1/1(delta_steerwheel [deg]) -> Dynamics_Simple/1(DeltaSteer_[deg]), [delta]
  Dynamics_Simple/1(State) -> STATE_Audi_A8_1/1, [human_view]
  Antenna_Rx_1_BusSelector/16 -> EEB/22(CAM_rotZ_in)  "<rotZ>"
  Antenna_Rx_1_BusSelector/15 -> EEB/21(CAM_GPSalt_in)  "<GPS_alt>"
  Antenna_Rx_1_BusSelector/14 -> EEB/20(CAM_GPSlong_in)  "<GPS_long>"
  Antenna_Rx_1_BusSelector/13 -> EEB/19(CAM_GPSlat_in)  "<GPS_lat>"
  Antenna_Rx_1_BusSelector/12 -> EEB/18(CAM_trafficLightPriority_in)  "<trafficLightPriority>"
  Antenna_Rx_1_BusSelector/11 -> EEB/17(CAM_turnAdvice_in)  "<turnAdvice>"
  Antenna_Rx_1_BusSelector/10 -> EEB/16(CAM_yawRate_in)  "<yawRate>"
  Antenna_Rx_1_BusSelector/9 -> EEB/15(CAM_acceleration_in)  "<acceleration>"
  Antenna_Rx_1_BusSelector/8 -> EEB/14(CAM_velocity_in)  "<velocity>"
  Antenna_Rx_1_BusSelector/7 -> EEB/13(CAM_sireneInUse_in)  "<sireneInUse>"
  Antenna_Rx_1_BusSelector/6 -> EEB/12(CAM_lightBarInUse_in)  "<lightBarInUse>"
  Antenna_Rx_1_BusSelector/5 -> EEB/11(CAM_publicVehicleType_in)  "<publicVehicleType>"
  Antenna_Rx_1_BusSelector/4 -> EEB/10(CAM_vehicleType_in)  "<actorType>"
  Antenna_Rx_1_BusSelector/3 -> EEB/9(CAM_vehicleID_in)  "<actorID>"
  Antenna_Rx_1_BusSelector/2 -> EEB/8(CAM_messageID_in)  "<messageID>"
  Antenna_Rx_1_BusSelector/1 -> EEB/7(CAM_warning_in)  "<warning>"
  SELF_Demux/9(GPS alt [m]) -> EEB/3(selfGPSAltitude)
  SELF_Demux/8(GPS long [deg]) -> EEB/2(selfGPSLongitude)
  SELF_Demux/7(GPS lat [deg]) -> EEB/1(selfGPSLatitude)
  PathFollower_1/3(brake pressure [bar]) -> Dynamics_Simple/3(Brake), [Brake]
  PathFollower_1/2(throttle [%]) -> Dynamics_Simple/2(Throttle), [Throttle]
  SELF_Demux/12(yaw rate [deg/s]) -> EEB/6(selfYawRate)
  SELF_Demux/5(roty [deg]) -> [rotY_deg]
  wheel Z disp/4(zDisp RR [m]) -> VISUWheels_Mux/7(zDisp RR [m])
  wheel Z disp/3(zDisp RL [m]) -> VISUWheels_Mux/6(zDisp RL [m])
  wheel Z disp/2(zDisp FR [m]) -> VISUWheels_Mux/5(zDisp FR [m])
  wheel Z disp/1(zDisp FL [m]) -> VISUWheels_Mux/4(zDisp FL [m])
  SELF_Demux/10(velocity [m/s]) -> PathFollower_1/6(velocity [m/s]), EEB/5(selfVelocity)
  SELF_Demux/6(rotz [deg]) -> Mux/3, EEB/4(selfRotZ)
  SELF_Demux/2(y [m]) -> Mux/2
  SELF_Demux/1(x [m]) -> Mux/1
  Mux/1 -> PathFollower_1/3(position x,y,Y [m,m,deg])
  V/1 -> PathFollower_1/4(Initial Velocity [m/s]), PathFollower_1/5(Desired Velocity [m/s])
  TextureColor1/1 -> Switch/1
  Switch/1 -> VISUTextureColor_Mux/1(RGB [-,-,-])
  Integer Delay6/1 -> Antenna_Tx_1_Mux/6(spare)
  Integer Delay2/1 -> VISUWheels_Mux/1(Steer Angle Front [deg])
  Dynamics_Simple/3(Perf_Params) -> [Params]
  Integer Delay3/1 -> VISUWheels_Mux/3(Velocity [m/s])
  Integer Delay4/1 -> VISULightSource_Mux/11(BrakeLightLeft), VISULightSource_Mux/12(BrakeLightRight)
  Integer Delay5/1 -> VISUSteer_Mux/2(Steer [deg])
  Antenna_Tx_1_BusAssignment/1 -> [Bus_Spare]
  Antenna_Rx_1_Demux/1(Vehicle_ID) -> Terminator_1/1
  Antenna_Rx_1_Demux/2(GPS_pos_lat_[deg]) -> Terminator_2/1
  Antenna_Rx_1_Demux/3(GPS_pos_long_[deg]) -> Terminator_3/1
  Antenna_Rx_1_Demux/4(GPS_pos_alt_[m]) -> Terminator_4/1
  Antenna_Rx_1_Demux/5(Velocity_[m/s]) -> Terminator_5/1
  Antenna_Rx_1_Demux/6(Acceleration_[m/s2]) -> Terminator_6/1
  Antenna_Rx_1_Demux/7(Heading [deg]) -> Terminator_7/1
  Antenna_Rx_1_Demux/8(warning_signal_id) -> Terminator_8/1
  Antenna_Rx_1_Demux/9(maneuvre_id) -> Terminator_9/1
  Antenna_Rx_1_Demux/10(vehicle_type) -> Terminator_10/1
  Antenna_Rx_1_Demux/11(brakingcapacity) -> Terminator_11/1
  Antenna_Rx_1_Demux/12(vehicle_size) -> Terminator_12/1
  Ground_1/1 -> Antenna_Tx_1_BusAssignment/2
  Ground_2/1 -> Antenna_Tx_1_BusAssignment/3
  Ground_3/1 -> Antenna_Tx_1_BusAssignment/4
  Ground_4/1 -> Antenna_Tx_1_BusAssignment/5
  Ground_5/1 -> Antenna_Tx_1_BusAssignment/6
  Ground_6/1 -> Antenna_Tx_1_BusAssignment/7
  Ground_7/1 -> Antenna_Tx_1_BusAssignment/8
  Ground_8/1 -> Antenna_Tx_1_BusAssignment/9
  Ground_9/1 -> Antenna_Tx_1_BusAssignment/10
  Ground_10/1 -> Antenna_Tx_1_BusAssignment/11
  Ground_11/1 -> Antenna_Tx_1_BusAssignment/12
  Ground_12/1 -> Antenna_Tx_1_BusAssignment/13
  Ground_13/1 -> Antenna_Tx_1_BusAssignment/14
  Ground_14/1 -> Antenna_Tx_1_BusAssignment/15
  Ground_15/1 -> Antenna_Tx_1_BusAssignment/16
  Ground_16/1 -> Antenna_Tx_1_BusAssignment/17
  Ground_17/1 -> Antenna_Tx_1_Mux/1(warning_signal_id)
  Ground_18/1 -> Antenna_Tx_1_Mux/2(maneuvre_id)
  Ground_19/1 -> Antenna_Tx_1_Mux/3(vehicle_type)
  Ground_20/1 -> Antenna_Tx_1_Mux/4(brakingcapacity)
  Ground_21/1 -> Antenna_Tx_1_Mux/5(vehicle_size)
  Ground_22/1 -> Dynamics_Simple/5(AutoManual_OnOff)
  Ground_23/1 -> Dynamics_Simple/7(Manual_GearShift)
  Ground_24/1 -> PathFollower_1/2(ActorOffset_Left(+) / Right(-) [m])
  PathFollower_1/6(Actor/Traj_distance [m]) -> Terminator_13/1
  PathFollower_1/7(Actor/Traj_angle [deg]) -> Terminator_14/1
  SELF_Demux/3(z [m]) -> Terminator_15/1
  SELF_Demux/4(rotx [deg]) -> Terminator_16/1
  SELF_Demux/11(heading [deg]) -> Terminator_17/1
  Trajectories/1(State) -> Terminator_18/1
  Ground_25/1 -> VISULightSource_Mux/1(IndicatorLightsLeft)
  Ground_26/1 -> VISULightSource_Mux/2(IndicatorLightsRight)
  Ground_27/1 -> VISULightSource_Mux/3(FogLightRearLeft)
  Ground_28/1 -> VISULightSource_Mux/4(FogLightRearRight)
  Ground_29/1 -> VISULightSource_Mux/5(FogLightFrontLeft)
  Ground_30/1 -> VISULightSource_Mux/6(FogLightFrontRight)
  Ground_31/1 -> VISULightSource_Mux/7(MainLightRearLeft)
  Ground_32/1 -> VISULightSource_Mux/8(MainLightRearRight)
  Ground_33/1 -> VISULightSource_Mux/9(MainLightFrontLeft)
  Ground_34/1 -> VISULightSource_Mux/10(MainLightFrontRight)
  Ground_35/1 -> VISUSteer_Mux/1(Column [deg])
  Ground_36/1 -> VISUWheels_Mux/2(Steer Angle Rear [deg])
